simulink library "AtomicLibrary"
PostLoadFcn:
  | PacketBusGenerator; RailCabBusGenerator
(part 2 of 8)

== system AtomicLibrary/UserInterface/Link Layer STATUS.slave ==
  port_in : Inport  Tag=id=_sTPDcPdmEeGH_6eRdlYQdA  Port=1  PortDimensions=-1  DataType=auto  OutDataType=fixdt(1, 16)  OutScaling=2^0  UseBusObject=on  OutDataTypeStr=Inherit: auto
      settings: BusObject=PacketBus
  net_address : Inport  Tag=id=_sTW_QPdmEeGH_6eRdlYQdA  Port=2  PortDimensions=-1  DataType=uint8  OutDataType=fixdt(1, 16)  OutScaling=2^0  OutDataTypeStr=uint8
  receiver_net_address : Inport  Tag=id=_sTXmUPdmEeGH_6eRdlYQdA  Port=3  PortDimensions=-1  DataType=uint8  OutDataType=fixdt(1, 16)  OutScaling=2^0  OutDataTypeStr=uint8
  read_event_queue_in : Inport  Tag=id=_sTQRkPdmEeGH_6eRdlYQdA  Port=4  PortDimensions=-1  DataType=auto  OutDataType=fixdt(1, 16)  OutScaling=2^0  OutDataTypeStr=Inherit: auto
  read_event_param_queue_in : Inport  Tag=id=_sTSt0PdmEeGH_6eRdlYQdA  Port=5  PortDimensions=-1  DataType=auto  OutDataType=fixdt(1, 16)  OutScaling=2^0  OutDataTypeStr=Inherit: auto
  read_event_queue_out : Inport  Tag=id=_sTT78PdmEeGH_6eRdlYQdA  Port=6  PortDimensions=-1  DataType=auto  OutDataType=fixdt(1, 16)  OutScaling=2^0  OutDataTypeStr=Inherit: auto
  read_event_param_queue_out : Inport  Tag=id=_sTUjAPdmEeGH_6eRdlYQdA  Port=7  PortDimensions=-1  DataType=auto  OutDataType=fixdt(1, 16)  OutScaling=2^0  OutDataTypeStr=Inherit: auto
  port_out : Outport  Tag=id=_sTN1UPdmEeGH_6eRdlYQdA  Port=1  PortDimensions=-1  DataType=auto  OutDataType=fixdt(1, 16)  OutScaling=2^0  UseBusObject=on  OutDataTypeStr=Inherit: auto
      settings: BusObject=PacketBus
  write_event_queue_in : Outport  Tag=id=_sTRfsPdmEeGH_6eRdlYQdA  Port=2  PortDimensions=-1  DataType=auto  OutDataType=fixdt(1, 16)  OutScaling=2^0  OutDataTypeStr=Inherit: auto
  write_event_param_queue_in : Outport  Tag=id=_sTSGwPdmEeGH_6eRdlYQdA  Port=3  PortDimensions=-1  DataType=auto  OutDataType=fixdt(1, 16)  OutScaling=2^0  OutDataTypeStr=Inherit: auto
  write_event_queue_out : Outport  Tag=id=_sTVKEPdmEeGH_6eRdlYQdA  Port=4  PortDimensions=-1  DataType=auto  OutDataType=fixdt(1, 16)  OutScaling=2^0  OutDataTypeStr=Inherit: auto
  write_event_param_queue_out : Outport  Tag=id=_sTWYMPdmEeGH_6eRdlYQdA  Port=5  PortDimensions=-1  DataType=auto  OutDataType=fixdt(1, 16)  OutScaling=2^0  OutDataTypeStr=Inherit: auto
  DataLinkLayer : Subsystem  Tag=id=_sTZbgfdmEeGH_6eRdlYQdA
  Bus Selector : BusSelector  OutputSignals=from,to,msg,param,pkgid,time  Tag=id=_sTY0cPdmEeGH_6eRdlYQdA
  Unit Delay1 : UnitDelay  Tag=id=_sTY0cfdmEeGH_6eRdlYQdA  SampleTime=-1
  Unit Delay2 : UnitDelay  Tag=id=_sTZbgPdmEeGH_6eRdlYQdA  SampleTime=-1
  Unit Delay3 : UnitDelay  Tag=id=_sTZbgvdmEeGH_6eRdlYQdA  SampleTime=-1
  Bus Creator : BusCreator  Inputs=6  UseBusObject=on  Tag=id=_sTaCkPdmEeGH_6eRdlYQdA
      settings: BusObject=PacketBus
  Unit Delay4 : UnitDelay  Tag=id=_sTaCkfdmEeGH_6eRdlYQdA  SampleTime=-1
  Terminator : Terminator
      settings: Tag=id=_sTapoPdmEeGH_6eRdlYQdA
  Receive Packet : Stateflow chart  Tag=id=_sTapofdmEeGH_6eRdlYQdA
  Send Packet : Stateflow chart  Tag=id=_sTbQsPdmEeGH_6eRdlYQdA
  wires:
  DataLinkLayer/3(snd_msg_out) -> Bus Creator/3
  DataLinkLayer/8(recv_msg_out) -> Receive Packet/2(packetMsg)
  Send Packet/3(eventQueue) -> Unit Delay1/1
  DataLinkLayer/7(recv_from_out) -> Receive Packet/1(packetFrom)
  Bus Selector/3 -> DataLinkLayer/3(recv_msg_in)
  read_event_param_queue_in/1 -> Receive Packet/5(eventParamQueueIn)
  Receive Packet/3(bufferOverflow) -> Terminator/1
  receiver_net_address/1 -> DataLinkLayer/8(snd_to_in)
  Receive Packet/2(eventParamQueue) -> Unit Delay4/1
  read_event_queue_out/1 -> Send Packet/2(eventQueueIn)
  DataLinkLayer/9(recv_param_out) -> Receive Packet/3(packetParam)
  Send Packet/2(packetParam) -> DataLinkLayer/10(snd_param_in)
  Bus Selector/2 -> DataLinkLayer/2(recv_to_in)
  port_in/1 -> Bus Selector/1
  read_event_param_queue_out/1 -> Send Packet/3(eventParamQueueIn)
  Send Packet/4(eventParamQueue) -> Unit Delay2/1
  Bus Selector/5 -> DataLinkLayer/5(recv_pkgid_in)
  Unit Delay4/1 -> write_event_param_queue_in/1
  read_event_queue_in/1 -> Receive Packet/4(eventQueueIn)
  Bus Selector/4 -> DataLinkLayer/4(recv_param_in)
  DataLinkLayer/2(snd_to_out) -> Bus Creator/2
  Bus Selector/6 -> DataLinkLayer/6(recv_time_in), Send Packet/1(busSizeSignal)
  Receive Packet/1(eventQueue) -> Unit Delay3/1
  DataLinkLayer/6(snd_time_out) -> Bus Creator/6
  Unit Delay1/1 -> write_event_queue_out/1
  DataLinkLayer/1(snd_from_out) -> Bus Creator/1
  DataLinkLayer/5(snd_pkgid_out) -> Bus Creator/5
  net_address/1 -> DataLinkLayer/7(snd_from_in)
  Send Packet/1(packetMsg) -> DataLinkLayer/9(snd_msg_in)
  Bus Creator/1 -> port_out/1  "Outport17"
  Unit Delay3/1 -> write_event_queue_in/1
  Bus Selector/1 -> DataLinkLayer/1(recv_from_in)
  Unit Delay2/1 -> write_event_param_queue_out/1
  DataLinkLayer/4(snd_param_out) -> Bus Creator/4

== system AtomicLibrary/UserInterface/Link Layer HMI_END.master ==
  port_in : Inport  Tag=id=_sdXP0PdmEeGH_6eRdlYQdA  Port=1  PortDimensions=-1  DataType=auto  OutDataType=fixdt(1, 16)  OutScaling=2^0  UseBusObject=on  OutDataTypeStr=Inherit: auto
      settings: BusObject=PacketBus
  net_address : Inport  Tag=id=_sdd9gPdmEeGH_6eRdlYQdA  Port=2  PortDimensions=-1  DataType=uint8  OutDataType=fixdt(1, 16)  OutScaling=2^0  OutDataTypeStr=uint8
  receiver_net_address : Inport  Tag=id=_sdekkPdmEeGH_6eRdlYQdA  Port=3  PortDimensions=-1  DataType=uint8  OutDataType=fixdt(1, 16)  OutScaling=2^0  OutDataTypeStr=uint8
  read_event_queue_in : Inport  Tag=id=_sdX24PdmEeGH_6eRdlYQdA  Port=4  PortDimensions=-1  DataType=auto  OutDataType=fixdt(1, 16)  OutScaling=2^0  OutDataTypeStr=Inherit: auto
  read_event_param_queue_in : Inport  Tag=id=_sdaTIPdmEeGH_6eRdlYQdA  Port=5  PortDimensions=-1  DataType=auto  OutDataType=fixdt(1, 16)  OutScaling=2^0  OutDataTypeStr=Inherit: auto
  read_event_queue_out : Inport  Tag=id=_sda6MPdmEeGH_6eRdlYQdA  Port=6  PortDimensions=-1  DataType=auto  OutDataType=fixdt(1, 16)  OutScaling=2^0  OutDataTypeStr=Inherit: auto
  read_event_param_queue_out : Inport  Tag=id=_sdbhQPdmEeGH_6eRdlYQdA  Port=7  PortDimensions=-1  DataType=auto  OutDataType=fixdt(1, 16)  OutScaling=2^0  OutDataTypeStr=Inherit: auto
  port_out : Outport  Tag=id=_sdWBsfdmEeGH_6eRdlYQdA  Port=1  PortDimensions=-1  DataType=auto  OutDataType=fixdt(1, 16)  OutScaling=2^0  UseBusObject=on  OutDataTypeStr=Inherit: auto
      settings: BusObject=PacketBus
  write_event_queue_in : Outport  Tag=id=_sdYd8PdmEeGH_6eRdlYQdA  Port=2  PortDimensions=-1  DataType=auto  OutDataType=fixdt(1, 16)  OutScaling=2^0  OutDataTypeStr=Inherit: auto
  write_event_param_queue_in : Outport  Tag=id=_sdZFAPdmEeGH_6eRdlYQdA  Port=3  PortDimensions=-1  DataType=auto  OutDataType=fixdt(1, 16)  OutScaling=2^0  OutDataTypeStr=Inherit: auto
  write_event_queue_out : Outport  Tag=id=_sdcIUPdmEeGH_6eRdlYQdA  Port=4  PortDimensions=-1  DataType=auto  OutDataType=fixdt(1, 16)  OutScaling=2^0  OutDataTypeStr=Inherit: auto
  write_event_param_queue_out : Outport  Tag=id=_sddWcPdmEeGH_6eRdlYQdA  Port=5  PortDimensions=-1  DataType=auto  OutDataType=fixdt(1, 16)  OutScaling=2^0  OutDataTypeStr=Inherit: auto
  DataLinkLayer : Subsystem  Tag=id=_sdgZwfdmEeGH_6eRdlYQdA
  Bus Selector : BusSelector  OutputSignals=from,to,msg,param,pkgid,time  Tag=id=_sdfysPdmEeGH_6eRdlYQdA
  Unit Delay1 : UnitDelay  Tag=id=_sdfysfdmEeGH_6eRdlYQdA  SampleTime=-1
  Unit Delay2 : UnitDelay  Tag=id=_sdgZwPdmEeGH_6eRdlYQdA  SampleTime=-1
  Unit Delay3 : UnitDelay  Tag=id=_sdhA0PdmEeGH_6eRdlYQdA  SampleTime=-1
  Bus Creator : BusCreator  Inputs=6  UseBusObject=on  Tag=id=_sdhA0fdmEeGH_6eRdlYQdA
      settings: BusObject=PacketBus
  Unit Delay4 : UnitDelay  Tag=id=_sdhA0vdmEeGH_6eRdlYQdA  SampleTime=-1
  Terminator : Terminator
      settings: Tag=id=_sdhn4PdmEeGH_6eRdlYQdA
  Receive Packet : Stateflow chart  Tag=id=_sdhn4fdmEeGH_6eRdlYQdA
  Send Packet : Stateflow chart  Tag=id=_sdiO8PdmEeGH_6eRdlYQdA
  wires:
  DataLinkLayer/3(snd_msg_out) -> Bus Creator/3
  DataLinkLayer/8(recv_msg_out) -> Receive Packet/2(packetMsg)
  Send Packet/3(eventQueue) -> Unit Delay1/1
  DataLinkLayer/7(recv_from_out) -> Receive Packet/1(packetFrom)
  Bus Selector/3 -> DataLinkLayer/3(recv_msg_in)
  read_event_param_queue_in/1 -> Receive Packet/5(eventParamQueueIn)
  Receive Packet/3(bufferOverflow) -> Terminator/1
  receiver_net_address/1 -> DataLinkLayer/8(snd_to_in)
  Receive Packet/2(eventParamQueue) -> Unit Delay4/1
  read_event_queue_out/1 -> Send Packet/2(eventQueueIn)
  DataLinkLayer/9(recv_param_out) -> Receive Packet/3(packetParam)
  Send Packet/2(packetParam) -> DataLinkLayer/10(snd_param_in)
  Bus Selector/2 -> DataLinkLayer/2(recv_to_in)
  port_in/1 -> Bus Selector/1
  read_event_param_queue_out/1 -> Send Packet/3(eventParamQueueIn)
  Send Packet/4(eventParamQueue) -> Unit Delay2/1
  Bus Selector/5 -> DataLinkLayer/5(recv_pkgid_in)
  Unit Delay4/1 -> write_event_param_queue_in/1
  read_event_queue_in/1 -> Receive Packet/4(eventQueueIn)
  Bus Selector/4 -> DataLinkLayer/4(recv_param_in)
  DataLinkLayer/2(snd_to_out) -> Bus Creator/2
  Bus Selector/6 -> DataLinkLayer/6(recv_time_in), Send Packet/1(busSizeSignal)
  Receive Packet/1(eventQueue) -> Unit Delay3/1
  DataLinkLayer/6(snd_time_out) -> Bus Creator/6
  Unit Delay1/1 -> write_event_queue_out/1
  DataLinkLayer/1(snd_from_out) -> Bus Creator/1
  DataLinkLayer/5(snd_pkgid_out) -> Bus Creator/5
  net_address/1 -> DataLinkLayer/7(snd_from_in)
  Send Packet/1(packetMsg) -> DataLinkLayer/9(snd_msg_in)
  Bus Creator/1 -> port_out/1  "Outport19"
  Unit Delay3/1 -> write_event_queue_in/1
  Bus Selector/1 -> DataLinkLayer/1(recv_from_in)
  Unit Delay2/1 -> write_event_param_queue_out/1
  DataLinkLayer/4(snd_param_out) -> Bus Creator/4

== system AtomicLibrary/TestDelegationSlave/Link Layer delegation_slave ==
  port_in : Inport  Tag=id=_qiNKsPdmEeGH_6eRdlYQdA  Port=1  PortDimensions=-1  DataType=auto  OutDataType=fixdt(1, 16)  OutScaling=2^0  UseBusObject=on  OutDataTypeStr=Inherit: auto
      settings: BusObject=PacketBus
  net_address : Inport  Tag=id=_qiT4YPdmEeGH_6eRdlYQdA  Port=2  PortDimensions=-1  DataType=uint8  OutDataType=fixdt(1, 16)  OutScaling=2^0  OutDataTypeStr=uint8
  receiver_net_address : Inport  Tag=id=_qiVGgPdmEeGH_6eRdlYQdA  Port=3  PortDimensions=-1  DataType=uint8  OutDataType=fixdt(1, 16)  OutScaling=2^0  OutDataTypeStr=uint8
  read_event_queue_in : Inport  Tag=id=_qiNxwPdmEeGH_6eRdlYQdA  Port=4  PortDimensions=-1  DataType=auto  OutDataType=fixdt(1, 16)  OutScaling=2^0  OutDataTypeStr=Inherit: auto
  read_event_param_queue_in : Inport  Tag=id=_qiQOAPdmEeGH_6eRdlYQdA  Port=5  PortDimensions=-1  DataType=auto  OutDataType=fixdt(1, 16)  OutScaling=2^0  OutDataTypeStr=Inherit: auto
  read_event_queue_out : Inport  Tag=id=_qiQ1EPdmEeGH_6eRdlYQdA  Port=6  PortDimensions=-1  DataType=auto  OutDataType=fixdt(1, 16)  OutScaling=2^0  OutDataTypeStr=Inherit: auto
  read_event_param_queue_out : Inport  Tag=id=_qiSDMPdmEeGH_6eRdlYQdA  Port=7  PortDimensions=-1  DataType=auto  OutDataType=fixdt(1, 16)  OutScaling=2^0  OutDataTypeStr=Inherit: auto
  port_out : Outport  Tag=id=_qiL8kfdmEeGH_6eRdlYQdA  Port=1  PortDimensions=-1  DataType=auto  OutDataType=fixdt(1, 16)  OutScaling=2^0  UseBusObject=on  OutDataTypeStr=Inherit: auto
      settings: BusObject=PacketBus
  write_event_queue_in : Outport  Tag=id=_qiO_4PdmEeGH_6eRdlYQdA  Port=2  PortDimensions=-1  DataType=auto  OutDataType=fixdt(1, 16)  OutScaling=2^0  OutDataTypeStr=Inherit: auto
  write_event_param_queue_in : Outport  Tag=id=_qiPm8PdmEeGH_6eRdlYQdA  Port=3  PortDimensions=-1  DataType=auto  OutDataType=fixdt(1, 16)  OutScaling=2^0  OutDataTypeStr=Inherit: auto
  write_event_queue_out : Outport  Tag=id=_qiSqQPdmEeGH_6eRdlYQdA  Port=4  PortDimensions=-1  DataType=auto  OutDataType=fixdt(1, 16)  OutScaling=2^0  OutDataTypeStr=Inherit: auto
  write_event_param_queue_out : Outport  Tag=id=_qiTRUPdmEeGH_6eRdlYQdA  Port=5  PortDimensions=-1  DataType=auto  OutDataType=fixdt(1, 16)  OutScaling=2^0  OutDataTypeStr=Inherit: auto
  DataLinkLayer : Subsystem  Tag=id=_qiW7sfdmEeGH_6eRdlYQdA
  Bus Selector : BusSelector  OutputSignals=from,to,msg,param,pkgid,time  Tag=id=_qiWUoPdmEeGH_6eRdlYQdA
  Unit Delay1 : UnitDelay  Tag=id=_qiWUofdmEeGH_6eRdlYQdA  SampleTime=-1
  Unit Delay2 : UnitDelay  Tag=id=_qiW7sPdmEeGH_6eRdlYQdA  SampleTime=-1
  Unit Delay3 : UnitDelay  Tag=id=_qiXiwPdmEeGH_6eRdlYQdA  SampleTime=-1
  Bus Creator : BusCreator  Inputs=6  UseBusObject=on  Tag=id=_qiYJ0PdmEeGH_6eRdlYQdA
      settings: BusObject=PacketBus
  Unit Delay4 : UnitDelay  Tag=id=_qiYw4PdmEeGH_6eRdlYQdA  SampleTime=-1
  Terminator : Terminator
      settings: Tag=id=_qillMPdmEeGH_6eRdlYQdA
  Receive Packet : Stateflow chart  Tag=id=_qimMQPdmEeGH_6eRdlYQdA
  Send Packet : Stateflow chart  Tag=id=_qimMQfdmEeGH_6eRdlYQdA
  wires:
  DataLinkLayer/3(snd_msg_out) -> Bus Creator/3
  DataLinkLayer/8(recv_msg_out) -> Receive Packet/2(packetMsg)
  Send Packet/3(eventQueue) -> Unit Delay1/1
  DataLinkLayer/7(recv_from_out) -> Receive Packet/1(packetFrom)
  Bus Selector/3 -> DataLinkLayer/3(recv_msg_in)
  read_event_param_queue_in/1 -> Receive Packet/5(eventParamQueueIn)
  Receive Packet/3(bufferOverflow) -> Terminator/1
  receiver_net_address/1 -> DataLinkLayer/8(snd_to_in)
  Receive Packet/2(eventParamQueue) -> Unit Delay4/1
  read_event_queue_out/1 -> Send Packet/2(eventQueueIn)
  DataLinkLayer/9(recv_param_out) -> Receive Packet/3(packetParam)
  Send Packet/2(packetParam) -> DataLinkLayer/10(snd_param_in)
  Bus Selector/2 -> DataLinkLayer/2(recv_to_in)
  port_in/1 -> Bus Selector/1
  read_event_param_queue_out/1 -> Send Packet/3(eventParamQueueIn)
  Send Packet/4(eventParamQueue) -> Unit Delay2/1
  Bus Selector/5 -> DataLinkLayer/5(recv_pkgid_in)
  Unit Delay4/1 -> write_event_param_queue_in/1
  read_event_queue_in/1 -> Receive Packet/4(eventQueueIn)
  Bus Selector/4 -> DataLinkLayer/4(recv_param_in)
  DataLinkLayer/2(snd_to_out) -> Bus Creator/2
  Bus Selector/6 -> DataLinkLayer/6(recv_time_in), Send Packet/1(busSizeSignal)
  Receive Packet/1(eventQueue) -> Unit Delay3/1
  DataLinkLayer/6(snd_time_out) -> Bus Creator/6
  Unit Delay1/1 -> write_event_queue_out/1
  DataLinkLayer/1(snd_from_out) -> Bus Creator/1
  DataLinkLayer/5(snd_pkgid_out) -> Bus Creator/5
  net_address/1 -> DataLinkLayer/7(snd_from_in)
  Send Packet/1(packetMsg) -> DataLinkLayer/9(snd_msg_in)
  Bus Creator/1 -> port_out/1  "Outport21"
  Unit Delay3/1 -> write_event_queue_in/1
  Bus Selector/1 -> DataLinkLayer/1(recv_from_in)
  Unit Delay2/1 -> write_event_param_queue_out/1
  DataLinkLayer/4(snd_param_out) -> Bus Creator/4

== system AtomicLibrary/TestDelegationMaster/Link Layer delegation_master ==
  port_in : Inport  Tag=id=_qrg3sPdmEeGH_6eRdlYQdA  Port=1  PortDimensions=-1  DataType=auto  OutDataType=fixdt(1, 16)  OutScaling=2^0  UseBusObject=on  OutDataTypeStr=Inherit: auto
      settings: BusObject=PacketBus
  net_address : Inport  Tag=id=_qrnlYPdmEeGH_6eRdlYQdA  Port=2  PortDimensions=-1  DataType=uint8  OutDataType=fixdt(1, 16)  OutScaling=2^0  OutDataTypeStr=uint8
  receiver_net_address : Inport  Tag=id=_qroMcPdmEeGH_6eRdlYQdA  Port=3  PortDimensions=-1  DataType=uint8  OutDataType=fixdt(1, 16)  OutScaling=2^0  OutDataTypeStr=uint8
  read_event_queue_in : Inport  Tag=id=_qrhewPdmEeGH_6eRdlYQdA  Port=4  PortDimensions=-1  DataType=auto  OutDataType=fixdt(1, 16)  OutScaling=2^0  OutDataTypeStr=Inherit: auto
  read_event_param_queue_in : Inport  Tag=id=_qrj7APdmEeGH_6eRdlYQdA  Port=5  PortDimensions=-1  DataType=auto  OutDataType=fixdt(1, 16)  OutScaling=2^0  OutDataTypeStr=Inherit: auto
  read_event_queue_out : Inport  Tag=id=_qrkiEPdmEeGH_6eRdlYQdA  Port=6  PortDimensions=-1  DataType=auto  OutDataType=fixdt(1, 16)  OutScaling=2^0  OutDataTypeStr=Inherit: auto
  read_event_param_queue_out : Inport  Tag=id=_qrlwMPdmEeGH_6eRdlYQdA  Port=7  PortDimensions=-1  DataType=auto  OutDataType=fixdt(1, 16)  OutScaling=2^0  OutDataTypeStr=Inherit: auto
  port_out : Outport  Tag=id=_qrgQofdmEeGH_6eRdlYQdA  Port=1  PortDimensions=-1  DataType=auto  OutDataType=fixdt(1, 16)  OutScaling=2^0  UseBusObject=on  OutDataTypeStr=Inherit: auto
      settings: BusObject=PacketBus
  write_event_queue_in : Outport  Tag=id=_qriF0PdmEeGH_6eRdlYQdA  Port=2  PortDimensions=-1  DataType=auto  OutDataType=fixdt(1, 16)  OutScaling=2^0  OutDataTypeStr=Inherit: auto
  write_event_param_queue_in : Outport  Tag=id=_qrjT8PdmEeGH_6eRdlYQdA  Port=3  PortDimensions=-1  DataType=auto  OutDataType=fixdt(1, 16)  OutScaling=2^0  OutDataTypeStr=Inherit: auto
  write_event_queue_out : Outport  Tag=id=_qrmXQPdmEeGH_6eRdlYQdA  Port=4  PortDimensions=-1  DataType=auto  OutDataType=fixdt(1, 16)  OutScaling=2^0  OutDataTypeStr=Inherit: auto
  write_event_param_queue_out : Outport  Tag=id=_qrm-UPdmEeGH_6eRdlYQdA  Port=5  PortDimensions=-1  DataType=auto  OutDataType=fixdt(1, 16)  OutScaling=2^0  OutDataTypeStr=Inherit: auto
  DataLinkLayer : Subsystem  Tag=id=_qrpakvdmEeGH_6eRdlYQdA
  Bus Selector : BusSelector  OutputSignals=from,to,msg,param,pkgid,time  Tag=id=_qrozgPdmEeGH_6eRdlYQdA
  Unit Delay1 : UnitDelay  Tag=id=_qrpakPdmEeGH_6eRdlYQdA  SampleTime=-1
  Unit Delay2 : UnitDelay  Tag=id=_qrpakfdmEeGH_6eRdlYQdA  SampleTime=-1
  Unit Delay3 : UnitDelay  Tag=id=_qrqBoPdmEeGH_6eRdlYQdA  SampleTime=-1
  Bus Creator : BusCreator  Inputs=6  UseBusObject=on  Tag=id=_qrqBofdmEeGH_6eRdlYQdA
      settings: BusObject=PacketBus
  Unit Delay4 : UnitDelay  Tag=id=_qrqosPdmEeGH_6eRdlYQdA  SampleTime=-1
  Terminator : Terminator
      settings: Tag=id=_qrqosfdmEeGH_6eRdlYQdA
  Receive Packet : Stateflow chart  Tag=id=_qrrPwPdmEeGH_6eRdlYQdA
  Send Packet : Stateflow chart  Tag=id=_qrrPwfdmEeGH_6eRdlYQdA
  wires:
  DataLinkLayer/3(snd_msg_out) -> Bus Creator/3
  DataLinkLayer/8(recv_msg_out) -> Receive Packet/2(packetMsg)
  Send Packet/3(eventQueue) -> Unit Delay1/1
  DataLinkLayer/7(recv_from_out) -> Receive Packet/1(packetFrom)
  Bus Selector/3 -> DataLinkLayer/3(recv_msg_in)
  read_event_param_queue_in/1 -> Receive Packet/5(eventParamQueueIn)
  Receive Packet/3(bufferOverflow) -> Terminator/1
  receiver_net_address/1 -> DataLinkLayer/8(snd_to_in)
  Receive Packet/2(eventParamQueue) -> Unit Delay4/1
  read_event_queue_out/1 -> Send Packet/2(eventQueueIn)
  DataLinkLayer/9(recv_param_out) -> Receive Packet/3(packetParam)
  Send Packet/2(packetParam) -> DataLinkLayer/10(snd_param_in)
  Bus Selector/2 -> DataLinkLayer/2(recv_to_in)
  port_in/1 -> Bus Selector/1
  read_event_param_queue_out/1 -> Send Packet/3(eventParamQueueIn)
  Send Packet/4(eventParamQueue) -> Unit Delay2/1
  Bus Selector/5 -> DataLinkLayer/5(recv_pkgid_in)
  Unit Delay4/1 -> write_event_param_queue_in/1
  read_event_queue_in/1 -> Receive Packet/4(eventQueueIn)
  Bus Selector/4 -> DataLinkLayer/4(recv_param_in)
  DataLinkLayer/2(snd_to_out) -> Bus Creator/2
  Bus Selector/6 -> DataLinkLayer/6(recv_time_in), Send Packet/1(busSizeSignal)
  Receive Packet/1(eventQueue) -> Unit Delay3/1
  DataLinkLayer/6(snd_time_out) -> Bus Creator/6
  Unit Delay1/1 -> write_event_queue_out/1
  DataLinkLayer/1(snd_from_out) -> Bus Creator/1
  DataLinkLayer/5(snd_pkgid_out) -> Bus Creator/5
  net_address/1 -> DataLinkLayer/7(snd_from_in)
  Send Packet/1(packetMsg) -> DataLinkLayer/9(snd_msg_in)
  Bus Creator/1 -> port_out/1  "Outport23"
  Unit Delay3/1 -> write_event_queue_in/1
  Bus Selector/1 -> DataLinkLayer/1(recv_from_in)
  Unit Delay2/1 -> write_event_param_queue_out/1
  DataLinkLayer/4(snd_param_out) -> Bus Creator/4

== system AtomicLibrary/TestEventListenerSlave/Link Layer eventListener_slave ==
  port_in : Inport  Tag=id=_q0oXcPdmEeGH_6eRdlYQdA  Port=1  PortDimensions=-1  DataType=auto  OutDataType=fixdt(1, 16)  OutScaling=2^0  UseBusObject=on  OutDataTypeStr=Inherit: auto
      settings: BusObject=PacketBus
  net_address : Inport  Tag=id=_q0vsMPdmEeGH_6eRdlYQdA  Port=2  PortDimensions=-1  DataType=uint8  OutDataType=fixdt(1, 16)  OutScaling=2^0  OutDataTypeStr=uint8
  receiver_net_address : Inport  Tag=id=_q0vsMfdmEeGH_6eRdlYQdA  Port=3  PortDimensions=-1  DataType=uint8  OutDataType=fixdt(1, 16)  OutScaling=2^0  OutDataTypeStr=uint8
  read_event_queue_in : Inport  Tag=id=_q0o-gPdmEeGH_6eRdlYQdA  Port=4  PortDimensions=-1  DataType=auto  OutDataType=fixdt(1, 16)  OutScaling=2^0  OutDataTypeStr=Inherit: auto
  read_event_param_queue_in : Inport  Tag=id=_q0rawPdmEeGH_6eRdlYQdA  Port=5  PortDimensions=-1  DataType=auto  OutDataType=fixdt(1, 16)  OutScaling=2^0  OutDataTypeStr=Inherit: auto
  read_event_queue_out : Inport  Tag=id=_q0so4PdmEeGH_6eRdlYQdA  Port=6  PortDimensions=-1  DataType=auto  OutDataType=fixdt(1, 16)  OutScaling=2^0  OutDataTypeStr=Inherit: auto
  read_event_param_queue_out : Inport  Tag=id=_q0tP8PdmEeGH_6eRdlYQdA  Port=7  PortDimensions=-1  DataType=auto  OutDataType=fixdt(1, 16)  OutScaling=2^0  OutDataTypeStr=Inherit: auto
  port_out : Outport  Tag=id=_q0nwYfdmEeGH_6eRdlYQdA  Port=1  PortDimensions=-1  DataType=auto  OutDataType=fixdt(1, 16)  OutScaling=2^0  UseBusObject=on  OutDataTypeStr=Inherit: auto
      settings: BusObject=PacketBus
  write_event_queue_in : Outport  Tag=id=_q0plkPdmEeGH_6eRdlYQdA  Port=2  PortDimensions=-1  DataType=auto  OutDataType=fixdt(1, 16)  OutScaling=2^0  OutDataTypeStr=Inherit: auto
  write_event_param_queue_in : Outport  Tag=id=_q0qzsPdmEeGH_6eRdlYQdA  Port=3  PortDimensions=-1  DataType=auto  OutDataType=fixdt(1, 16)  OutScaling=2^0  OutDataTypeStr=Inherit: auto
  write_event_queue_out : Outport  Tag=id=_q0t3APdmEeGH_6eRdlYQdA  Port=4  PortDimensions=-1  DataType=auto  OutDataType=fixdt(1, 16)  OutScaling=2^0  OutDataTypeStr=Inherit: auto
  write_event_param_queue_out : Outport  Tag=id=_q0ueEPdmEeGH_6eRdlYQdA  Port=5  PortDimensions=-1  DataType=auto  OutDataType=fixdt(1, 16)  OutScaling=2^0  OutDataTypeStr=Inherit: auto
  DataLinkLayer : Subsystem  Tag=id=_q0xhYPdmEeGH_6eRdlYQdA
  Bus Selector : BusSelector  OutputSignals=from,to,msg,param,pkgid,time  Tag=id=_q0w6UPdmEeGH_6eRdlYQdA
  Unit Delay1 : UnitDelay  Tag=id=_q0w6UfdmEeGH_6eRdlYQdA  SampleTime=-1
  Unit Delay2 : UnitDelay  Tag=id=_q0w6UvdmEeGH_6eRdlYQdA  SampleTime=-1
  Unit Delay3 : UnitDelay  Tag=id=_q0xhYfdmEeGH_6eRdlYQdA  SampleTime=-1
  Bus Creator : BusCreator  Inputs=6  UseBusObject=on  Tag=id=_q0yIcPdmEeGH_6eRdlYQdA
      settings: BusObject=PacketBus
  Unit Delay4 : UnitDelay  Tag=id=_q0yIcfdmEeGH_6eRdlYQdA  SampleTime=-1
  Terminator : Terminator
      settings: Tag=id=_q0yIcvdmEeGH_6eRdlYQdA
  Receive Packet : Stateflow chart  Tag=id=_q0yvgPdmEeGH_6eRdlYQdA
  Send Packet : Stateflow chart  Tag=id=_q0zWkPdmEeGH_6eRdlYQdA
  wires:
  DataLinkLayer/3(snd_msg_out) -> Bus Creator/3
  DataLinkLayer/8(recv_msg_out) -> Receive Packet/2(packetMsg)
  Send Packet/3(eventQueue) -> Unit Delay1/1
  DataLinkLayer/7(recv_from_out) -> Receive Packet/1(packetFrom)
  Bus Selector/3 -> DataLinkLayer/3(recv_msg_in)
  read_event_param_queue_in/1 -> Receive Packet/5(eventParamQueueIn)
  Receive Packet/3(bufferOverflow) -> Terminator/1
  receiver_net_address/1 -> DataLinkLayer/8(snd_to_in)
  Receive Packet/2(eventParamQueue) -> Unit Delay4/1
  read_event_queue_out/1 -> Send Packet/2(eventQueueIn)
  DataLinkLayer/9(recv_param_out) -> Receive Packet/3(packetParam)
  Send Packet/2(packetParam) -> DataLinkLayer/10(snd_param_in)
  Bus Selector/2 -> DataLinkLayer/2(recv_to_in)
  port_in/1 -> Bus Selector/1
  read_event_param_queue_out/1 -> Send Packet/3(eventParamQueueIn)
  Send Packet/4(eventParamQueue) -> Unit Delay2/1
  Bus Selector/5 -> DataLinkLayer/5(recv_pkgid_in)
  Unit Delay4/1 -> write_event_param_queue_in/1
  read_event_queue_in/1 -> Receive Packet/4(eventQueueIn)
  Bus Selector/4 -> DataLinkLayer/4(recv_param_in)
  DataLinkLayer/2(snd_to_out) -> Bus Creator/2
  Bus Selector/6 -> DataLinkLayer/6(recv_time_in), Send Packet/1(busSizeSignal)
  Receive Packet/1(eventQueue) -> Unit Delay3/1
  DataLinkLayer/6(snd_time_out) -> Bus Creator/6
  Unit Delay1/1 -> write_event_queue_out/1
  DataLinkLayer/1(snd_from_out) -> Bus Creator/1
  DataLinkLayer/5(snd_pkgid_out) -> Bus Creator/5
  net_address/1 -> DataLinkLayer/7(snd_from_in)
  Send Packet/1(packetMsg) -> DataLinkLayer/9(snd_msg_in)
  Bus Creator/1 -> port_out/1  "Outport25"
  Unit Delay3/1 -> write_event_queue_in/1
  Bus Selector/1 -> DataLinkLayer/1(recv_from_in)
  Unit Delay2/1 -> write_event_param_queue_out/1
  DataLinkLayer/4(snd_param_out) -> Bus Creator/4

== system AtomicLibrary/TestEventListenerMaster/Link Layer eventListener_master ==
  port_in : Inport  Tag=id=_q93L8PdmEeGH_6eRdlYQdA  Port=1  PortDimensions=-1  DataType=auto  OutDataType=fixdt(1, 16)  OutScaling=2^0  UseBusObject=on  OutDataTypeStr=Inherit: auto
      settings: BusObject=PacketBus
  net_address : Inport  Tag=id=_q99SkPdmEeGH_6eRdlYQdA  Port=2  PortDimensions=-1  DataType=uint8  OutDataType=fixdt(1, 16)  OutScaling=2^0  OutDataTypeStr=uint8
  receiver_net_address : Inport  Tag=id=_q995oPdmEeGH_6eRdlYQdA  Port=3  PortDimensions=-1  DataType=uint8  OutDataType=fixdt(1, 16)  OutScaling=2^0  OutDataTypeStr=uint8
  read_event_queue_in : Inport  Tag=id=_q93zAPdmEeGH_6eRdlYQdA  Port=4  PortDimensions=-1  DataType=auto  OutDataType=fixdt(1, 16)  OutScaling=2^0  OutDataTypeStr=Inherit: auto
  read_event_param_queue_in : Inport  Tag=id=_q96PQPdmEeGH_6eRdlYQdA  Port=5  PortDimensions=-1  DataType=auto  OutDataType=fixdt(1, 16)  OutScaling=2^0  OutDataTypeStr=Inherit: auto
  read_event_queue_out : Inport  Tag=id=_q962UPdmEeGH_6eRdlYQdA  Port=6  PortDimensions=-1  DataType=auto  OutDataType=fixdt(1, 16)  OutScaling=2^0  OutDataTypeStr=Inherit: auto
  read_event_param_queue_out : Inport  Tag=id=_q97dYPdmEeGH_6eRdlYQdA  Port=7  PortDimensions=-1  DataType=auto  OutDataType=fixdt(1, 16)  OutScaling=2^0  OutDataTypeStr=Inherit: auto
  port_out : Outport  Tag=id=_q92k4fdmEeGH_6eRdlYQdA  Port=1  PortDimensions=-1  DataType=auto  OutDataType=fixdt(1, 16)  OutScaling=2^0  UseBusObject=on  OutDataTypeStr=Inherit: auto
      settings: BusObject=PacketBus
  write_event_queue_in : Outport  Tag=id=_q94aEPdmEeGH_6eRdlYQdA  Port=2  PortDimensions=-1  DataType=auto  OutDataType=fixdt(1, 16)  OutScaling=2^0  OutDataTypeStr=Inherit: auto
  write_event_param_queue_in : Outport  Tag=id=_q95oMPdmEeGH_6eRdlYQdA  Port=3  PortDimensions=-1  DataType=auto  OutDataType=fixdt(1, 16)  OutScaling=2^0  OutDataTypeStr=Inherit: auto
  write_event_queue_out : Outport  Tag=id=_q98EcPdmEeGH_6eRdlYQdA  Port=4  PortDimensions=-1  DataType=auto  OutDataType=fixdt(1, 16)  OutScaling=2^0  OutDataTypeStr=Inherit: auto
  write_event_param_queue_out : Outport  Tag=id=_q98rgPdmEeGH_6eRdlYQdA  Port=5  PortDimensions=-1  DataType=auto  OutDataType=fixdt(1, 16)  OutScaling=2^0  OutDataTypeStr=Inherit: auto
  DataLinkLayer : Subsystem  Tag=id=_q9_HwvdmEeGH_6eRdlYQdA
  Bus Selector : BusSelector  OutputSignals=from,to,msg,param,pkgid,time  Tag=id=_q9-gsPdmEeGH_6eRdlYQdA
  Unit Delay1 : UnitDelay  Tag=id=_q9_HwPdmEeGH_6eRdlYQdA  SampleTime=-1
  Unit Delay2 : UnitDelay  Tag=id=_q9_HwfdmEeGH_6eRdlYQdA  SampleTime=-1
  Unit Delay3 : UnitDelay  Tag=id=_q9_u0PdmEeGH_6eRdlYQdA  SampleTime=-1
  Bus Creator : BusCreator  Inputs=6  UseBusObject=on  Tag=id=_q9_u0fdmEeGH_6eRdlYQdA
      settings: BusObject=PacketBus
  Unit Delay4 : UnitDelay  Tag=id=_q-AV4PdmEeGH_6eRdlYQdA  SampleTime=-1
  Terminator : Terminator
      settings: Tag=id=_q-AV4fdmEeGH_6eRdlYQdA
  Receive Packet : Stateflow chart  Tag=id=_q-AV4vdmEeGH_6eRdlYQdA
  Send Packet : Stateflow chart  Tag=id=_q-A88PdmEeGH_6eRdlYQdA
  wires:
  DataLinkLayer/3(snd_msg_out) -> Bus Creator/3
  DataLinkLayer/8(recv_msg_out) -> Receive Packet/2(packetMsg)
  Send Packet/3(eventQueue) -> Unit Delay1/1
  DataLinkLayer/7(recv_from_out) -> Receive Packet/1(packetFrom)
  Bus Selector/3 -> DataLinkLayer/3(recv_msg_in)
  read_event_param_queue_in/1 -> Receive Packet/5(eventParamQueueIn)
  Receive Packet/3(bufferOverflow) -> Terminator/1
  receiver_net_address/1 -> DataLinkLayer/8(snd_to_in)
  Receive Packet/2(eventParamQueue) -> Unit Delay4/1
  read_event_queue_out/1 -> Send Packet/2(eventQueueIn)
  DataLinkLayer/9(recv_param_out) -> Receive Packet/3(packetParam)
  Send Packet/2(packetParam) -> DataLinkLayer/10(snd_param_in)
  Bus Selector/2 -> DataLinkLayer/2(recv_to_in)
  port_in/1 -> Bus Selector/1
  read_event_param_queue_out/1 -> Send Packet/3(eventParamQueueIn)
  Send Packet/4(eventParamQueue) -> Unit Delay2/1
  Bus Selector/5 -> DataLinkLayer/5(recv_pkgid_in)
  Unit Delay4/1 -> write_event_param_queue_in/1
  read_event_queue_in/1 -> Receive Packet/4(eventQueueIn)
  Bus Selector/4 -> DataLinkLayer/4(recv_param_in)
  DataLinkLayer/2(snd_to_out) -> Bus Creator/2
  Bus Selector/6 -> DataLinkLayer/6(recv_time_in), Send Packet/1(busSizeSignal)
  Receive Packet/1(eventQueue) -> Unit Delay3/1
  DataLinkLayer/6(snd_time_out) -> Bus Creator/6
  Unit Delay1/1 -> write_event_queue_out/1
  DataLinkLayer/1(snd_from_out) -> Bus Creator/1
  DataLinkLayer/5(snd_pkgid_out) -> Bus Creator/5
  net_address/1 -> DataLinkLayer/7(snd_from_in)
  Send Packet/1(packetMsg) -> DataLinkLayer/9(snd_msg_in)
  Bus Creator/1 -> port_out/1  "Outport27"
  Unit Delay3/1 -> write_event_queue_in/1
  Bus Selector/1 -> DataLinkLayer/1(recv_from_in)
  Unit Delay2/1 -> write_event_param_queue_out/1
  DataLinkLayer/4(snd_param_out) -> Bus Creator/4

== system AtomicLibrary/TestTurnTransmission/Link Layer turn_transmission_partner ==
  port_in : Inport  Tag=id=_rGp7kPdmEeGH_6eRdlYQdA  Port=1  PortDimensions=-1  DataType=auto  OutDataType=fixdt(1, 16)  OutScaling=2^0  UseBusObject=on  OutDataTypeStr=Inherit: auto
      settings: BusObject=PacketBus
  net_address : Inport  Tag=id=_rGvbIPdmEeGH_6eRdlYQdA  Port=2  PortDimensions=-1  DataType=uint8  OutDataType=fixdt(1, 16)  OutScaling=2^0  OutDataTypeStr=uint8
  receiver_net_address : Inport  Tag=id=_rGwCMPdmEeGH_6eRdlYQdA  Port=3  PortDimensions=-1  DataType=uint8  OutDataType=fixdt(1, 16)  OutScaling=2^0  OutDataTypeStr=uint8
  read_event_queue_in : Inport  Tag=id=_rGqioPdmEeGH_6eRdlYQdA  Port=4  PortDimensions=-1  DataType=auto  OutDataType=fixdt(1, 16)  OutScaling=2^0  OutDataTypeStr=Inherit: auto
  read_event_param_queue_in : Inport  Tag=id=_rGsX0PdmEeGH_6eRdlYQdA  Port=5  PortDimensions=-1  DataType=auto  OutDataType=fixdt(1, 16)  OutScaling=2^0  OutDataTypeStr=Inherit: auto
  read_event_queue_out : Inport  Tag=id=_rGs-4PdmEeGH_6eRdlYQdA  Port=6  PortDimensions=-1  DataType=auto  OutDataType=fixdt(1, 16)  OutScaling=2^0  OutDataTypeStr=Inherit: auto
  read_event_param_queue_out : Inport  Tag=id=_rGtl8PdmEeGH_6eRdlYQdA  Port=7  PortDimensions=-1  DataType=auto  OutDataType=fixdt(1, 16)  OutScaling=2^0  OutDataTypeStr=Inherit: auto
  port_out : Outport  Tag=id=_rGpUgPdmEeGH_6eRdlYQdA  Port=1  PortDimensions=-1  DataType=auto  OutDataType=fixdt(1, 16)  OutScaling=2^0  UseBusObject=on  OutDataTypeStr=Inherit: auto
      settings: BusObject=PacketBus
  write_event_queue_in : Outport  Tag=id=_rGrJsPdmEeGH_6eRdlYQdA  Port=2  PortDimensions=-1  DataType=auto  OutDataType=fixdt(1, 16)  OutScaling=2^0  OutDataTypeStr=Inherit: auto
  write_event_param_queue_in : Outport  Tag=id=_rGrwwPdmEeGH_6eRdlYQdA  Port=3  PortDimensions=-1  DataType=auto  OutDataType=fixdt(1, 16)  OutScaling=2^0  OutDataTypeStr=Inherit: auto
  write_event_queue_out : Outport  Tag=id=_rGuNAPdmEeGH_6eRdlYQdA  Port=4  PortDimensions=-1  DataType=auto  OutDataType=fixdt(1, 16)  OutScaling=2^0  OutDataTypeStr=Inherit: auto
  write_event_param_queue_out : Outport  Tag=id=_rGu0EPdmEeGH_6eRdlYQdA  Port=5  PortDimensions=-1  DataType=auto  OutDataType=fixdt(1, 16)  OutScaling=2^0  OutDataTypeStr=Inherit: auto
  DataLinkLayer : Subsystem  Tag=id=_rGxQUvdmEeGH_6eRdlYQdA
  Bus Selector : BusSelector  OutputSignals=from,to,msg,param,pkgid,time  Tag=id=_rGwpQPdmEeGH_6eRdlYQdA
  Unit Delay1 : UnitDelay  Tag=id=_rGxQUPdmEeGH_6eRdlYQdA  SampleTime=-1
  Unit Delay2 : UnitDelay  Tag=id=_rGxQUfdmEeGH_6eRdlYQdA  SampleTime=-1
  Unit Delay3 : UnitDelay  Tag=id=_rGx3YPdmEeGH_6eRdlYQdA  SampleTime=-1
  Bus Creator : BusCreator  Inputs=6  UseBusObject=on  Tag=id=_rGx3YfdmEeGH_6eRdlYQdA
      settings: BusObject=PacketBus
  Unit Delay4 : UnitDelay  Tag=id=_rGyecPdmEeGH_6eRdlYQdA  SampleTime=-1
  Terminator : Terminator
      settings: Tag=id=_rGyecfdmEeGH_6eRdlYQdA
  Receive Packet : Stateflow chart  Tag=id=_rGzFgPdmEeGH_6eRdlYQdA
  Send Packet : Stateflow chart  Tag=id=_rGzFgfdmEeGH_6eRdlYQdA
  wires:
  DataLinkLayer/3(snd_msg_out) -> Bus Creator/3
  DataLinkLayer/8(recv_msg_out) -> Receive Packet/2(packetMsg)
  Send Packet/3(eventQueue) -> Unit Delay1/1
  DataLinkLayer/7(recv_from_out) -> Receive Packet/1(packetFrom)
  Bus Selector/3 -> DataLinkLayer/3(recv_msg_in)
  read_event_param_queue_in/1 -> Receive Packet/5(eventParamQueueIn)
  Receive Packet/3(bufferOverflow) -> Terminator/1
  receiver_net_address/1 -> DataLinkLayer/8(snd_to_in)
  Receive Packet/2(eventParamQueue) -> Unit Delay4/1
  read_event_queue_out/1 -> Send Packet/2(eventQueueIn)
  DataLinkLayer/9(recv_param_out) -> Receive Packet/3(packetParam)
  Send Packet/2(packetParam) -> DataLinkLayer/10(snd_param_in)
  Bus Selector/2 -> DataLinkLayer/2(recv_to_in)
  port_in/1 -> Bus Selector/1
  read_event_param_queue_out/1 -> Send Packet/3(eventParamQueueIn)
  Send Packet/4(eventParamQueue) -> Unit Delay2/1
  Bus Selector/5 -> DataLinkLayer/5(recv_pkgid_in)
  Unit Delay4/1 -> write_event_param_queue_in/1
  read_event_queue_in/1 -> Receive Packet/4(eventQueueIn)
  Bus Selector/4 -> DataLinkLayer/4(recv_param_in)
  DataLinkLayer/2(snd_to_out) -> Bus Creator/2
  Bus Selector/6 -> DataLinkLayer/6(recv_time_in), Send Packet/1(busSizeSignal)
  Receive Packet/1(eventQueue) -> Unit Delay3/1
  DataLinkLayer/6(snd_time_out) -> Bus Creator/6
  Unit Delay1/1 -> write_event_queue_out/1
  DataLinkLayer/1(snd_from_out) -> Bus Creator/1
  DataLinkLayer/5(snd_pkgid_out) -> Bus Creator/5
  net_address/1 -> DataLinkLayer/7(snd_from_in)
  Send Packet/1(packetMsg) -> DataLinkLayer/9(snd_msg_in)
  Bus Creator/1 -> port_out/1  "Outport29"
  Unit Delay3/1 -> write_event_queue_in/1
  Bus Selector/1 -> DataLinkLayer/1(recv_from_in)
  Unit Delay2/1 -> write_event_param_queue_out/1
  DataLinkLayer/4(snd_param_out) -> Bus Creator/4

== system AtomicLibrary/TestRequestInformationProvider/Link Layer requestinformation_provider ==
  port_in : Inport  Tag=id=_rPz3kPdmEeGH_6eRdlYQdA  Port=1  PortDimensions=-1  DataType=auto  OutDataType=fixdt(1, 16)  OutScaling=2^0  UseBusObject=on  OutDataTypeStr=Inherit: auto
      settings: BusObject=PacketBus
  net_address : Inport  Tag=id=_rP7zYPdmEeGH_6eRdlYQdA  Port=2  PortDimensions=-1  DataType=uint8  OutDataType=fixdt(1, 16)  OutScaling=2^0  OutDataTypeStr=uint8
  receiver_net_address : Inport  Tag=id=_rP8acPdmEeGH_6eRdlYQdA  Port=3  PortDimensions=-1  DataType=uint8  OutDataType=fixdt(1, 16)  OutScaling=2^0  OutDataTypeStr=uint8
  read_event_queue_in : Inport  Tag=id=_rP1FsPdmEeGH_6eRdlYQdA  Port=4  PortDimensions=-1  DataType=auto  OutDataType=fixdt(1, 16)  OutScaling=2^0  OutDataTypeStr=Inherit: auto
  read_event_param_queue_in : Inport  Tag=id=_rP4JAPdmEeGH_6eRdlYQdA  Port=5  PortDimensions=-1  DataType=auto  OutDataType=fixdt(1, 16)  OutScaling=2^0  OutDataTypeStr=Inherit: auto
  read_event_queue_out : Inport  Tag=id=_rP4wEPdmEeGH_6eRdlYQdA  Port=6  PortDimensions=-1  DataType=auto  OutDataType=fixdt(1, 16)  OutScaling=2^0  OutDataTypeStr=Inherit: auto
  read_event_param_queue_out : Inport  Tag=id=_rP5XIPdmEeGH_6eRdlYQdA  Port=7  PortDimensions=-1  DataType=auto  OutDataType=fixdt(1, 16)  OutScaling=2^0  OutDataTypeStr=Inherit: auto
  port_out : Outport  Tag=id=_rPzQgPdmEeGH_6eRdlYQdA  Port=1  PortDimensions=-1  DataType=auto  OutDataType=fixdt(1, 16)  OutScaling=2^0  UseBusObject=on  OutDataTypeStr=Inherit: auto
      settings: BusObject=PacketBus
  write_event_queue_in : Outport  Tag=id=_rP2T0PdmEeGH_6eRdlYQdA  Port=2  PortDimensions=-1  DataType=auto  OutDataType=fixdt(1, 16)  OutScaling=2^0  OutDataTypeStr=Inherit: auto
  write_event_param_queue_in : Outport  Tag=id=_rP264PdmEeGH_6eRdlYQdA  Port=3  PortDimensions=-1  DataType=auto  OutDataType=fixdt(1, 16)  OutScaling=2^0  OutDataTypeStr=Inherit: auto
  write_event_queue_out : Outport  Tag=id=_rP5-MPdmEeGH_6eRdlYQdA  Port=4  PortDimensions=-1  DataType=auto  OutDataType=fixdt(1, 16)  OutScaling=2^0  OutDataTypeStr=Inherit: auto
  write_event_param_queue_out : Outport  Tag=id=_rP7MUPdmEeGH_6eRdlYQdA  Port=5  PortDimensions=-1  DataType=auto  OutDataType=fixdt(1, 16)  OutScaling=2^0  OutDataTypeStr=Inherit: auto
  DataLinkLayer : Subsystem  Tag=id=_rP9okfdmEeGH_6eRdlYQdA
  Bus Selector : BusSelector  OutputSignals=from,to,msg,param,pkgid,time  Tag=id=_rP9BgPdmEeGH_6eRdlYQdA
  Unit Delay1 : UnitDelay  Tag=id=_rP9BgfdmEeGH_6eRdlYQdA  SampleTime=-1
  Unit Delay2 : UnitDelay  Tag=id=_rP9okPdmEeGH_6eRdlYQdA  SampleTime=-1
  Unit Delay3 : UnitDelay  Tag=id=_rP-PoPdmEeGH_6eRdlYQdA  SampleTime=-1
  Bus Creator : BusCreator  Inputs=6  UseBusObject=on  Tag=id=_rP-PofdmEeGH_6eRdlYQdA
      settings: BusObject=PacketBus
  Unit Delay4 : UnitDelay  Tag=id=_rP-PovdmEeGH_6eRdlYQdA  SampleTime=-1
  Terminator : Terminator
      settings: Tag=id=_rP-2sPdmEeGH_6eRdlYQdA
  Receive Packet : Stateflow chart  Tag=id=_rP-2sfdmEeGH_6eRdlYQdA
  Send Packet : Stateflow chart  Tag=id=_rP_dwPdmEeGH_6eRdlYQdA
  wires:
  DataLinkLayer/3(snd_msg_out) -> Bus Creator/3
  DataLinkLayer/8(recv_msg_out) -> Receive Packet/2(packetMsg)
  Send Packet/3(eventQueue) -> Unit Delay1/1
  DataLinkLayer/7(recv_from_out) -> Receive Packet/1(packetFrom)
  Bus Selector/3 -> DataLinkLayer/3(recv_msg_in)
  read_event_param_queue_in/1 -> Receive Packet/5(eventParamQueueIn)
  Receive Packet/3(bufferOverflow) -> Terminator/1
  receiver_net_address/1 -> DataLinkLayer/8(snd_to_in)
  Receive Packet/2(eventParamQueue) -> Unit Delay4/1
  read_event_queue_out/1 -> Send Packet/2(eventQueueIn)
  DataLinkLayer/9(recv_param_out) -> Receive Packet/3(packetParam)
  Send Packet/2(packetParam) -> DataLinkLayer/10(snd_param_in)
  Bus Selector/2 -> DataLinkLayer/2(recv_to_in)
  port_in/1 -> Bus Selector/1
  read_event_param_queue_out/1 -> Send Packet/3(eventParamQueueIn)
  Send Packet/4(eventParamQueue) -> Unit Delay2/1
  Bus Selector/5 -> DataLinkLayer/5(recv_pkgid_in)
  Unit Delay4/1 -> write_event_param_queue_in/1
  read_event_queue_in/1 -> Receive Packet/4(eventQueueIn)
  Bus Selector/4 -> DataLinkLayer/4(recv_param_in)
  DataLinkLayer/2(snd_to_out) -> Bus Creator/2
  Bus Selector/6 -> DataLinkLayer/6(recv_time_in), Send Packet/1(busSizeSignal)
  Receive Packet/1(eventQueue) -> Unit Delay3/1
  DataLinkLayer/6(snd_time_out) -> Bus Creator/6
  Unit Delay1/1 -> write_event_queue_out/1
  DataLinkLayer/1(snd_from_out) -> Bus Creator/1
  DataLinkLayer/5(snd_pkgid_out) -> Bus Creator/5
  net_address/1 -> DataLinkLayer/7(snd_from_in)
  Send Packet/1(packetMsg) -> DataLinkLayer/9(snd_msg_in)
  Bus Creator/1 -> port_out/1  "Outport31"
  Unit Delay3/1 -> write_event_queue_in/1
  Bus Selector/1 -> DataLinkLayer/1(recv_from_in)
  Unit Delay2/1 -> write_event_param_queue_out/1
  DataLinkLayer/4(snd_param_out) -> Bus Creator/4

== system AtomicLibrary/TestRequestInformaitonUser/Link Layer requestinformation_user ==
  port_in : Inport  Tag=id=_rYOzwPdmEeGH_6eRdlYQdA  Port=1  PortDimensions=-1  DataType=auto  OutDataType=fixdt(1, 16)  OutScaling=2^0  UseBusObject=on  OutDataTypeStr=Inherit: auto
      settings: BusObject=PacketBus
  net_address : Inport  Tag=id=_rYWvkPdmEeGH_6eRdlYQdA  Port=2  PortDimensions=-1  DataType=uint8  OutDataType=fixdt(1, 16)  OutScaling=2^0  OutDataTypeStr=uint8
  receiver_net_address : Inport  Tag=id=_rYX9sPdmEeGH_6eRdlYQdA  Port=3  PortDimensions=-1  DataType=uint8  OutDataType=fixdt(1, 16)  OutScaling=2^0  OutDataTypeStr=uint8
  read_event_queue_in : Inport  Tag=id=_rYPa0PdmEeGH_6eRdlYQdA  Port=4  PortDimensions=-1  DataType=auto  OutDataType=fixdt(1, 16)  OutScaling=2^0  OutDataTypeStr=Inherit: auto
  read_event_param_queue_in : Inport  Tag=id=_rYRQAPdmEeGH_6eRdlYQdA  Port=5  PortDimensions=-1  DataType=auto  OutDataType=fixdt(1, 16)  OutScaling=2^0  OutDataTypeStr=Inherit: auto
  read_event_queue_out : Inport  Tag=id=_rYSeIPdmEeGH_6eRdlYQdA  Port=6  PortDimensions=-1  DataType=auto  OutDataType=fixdt(1, 16)  OutScaling=2^0  OutDataTypeStr=Inherit: auto
  read_event_param_queue_out : Inport  Tag=id=_rYTsQPdmEeGH_6eRdlYQdA  Port=7  PortDimensions=-1  DataType=auto  OutDataType=fixdt(1, 16)  OutScaling=2^0  OutDataTypeStr=Inherit: auto
  port_out : Outport  Tag=id=_rYOMsPdmEeGH_6eRdlYQdA  Port=1  PortDimensions=-1  DataType=auto  OutDataType=fixdt(1, 16)  OutScaling=2^0  UseBusObject=on  OutDataTypeStr=Inherit: auto
      settings: BusObject=PacketBus
  write_event_queue_in : Outport  Tag=id=_rYQB4PdmEeGH_6eRdlYQdA  Port=2  PortDimensions=-1  DataType=auto  OutDataType=fixdt(1, 16)  OutScaling=2^0  OutDataTypeStr=Inherit: auto
  write_event_param_queue_in : Outport  Tag=id=_rYQo8PdmEeGH_6eRdlYQdA  Port=3  PortDimensions=-1  DataType=auto  OutDataType=fixdt(1, 16)  OutScaling=2^0  OutDataTypeStr=Inherit: auto
  write_event_queue_out : Outport  Tag=id=_rYUTUPdmEeGH_6eRdlYQdA  Port=4  PortDimensions=-1  DataType=auto  OutDataType=fixdt(1, 16)  OutScaling=2^0  OutDataTypeStr=Inherit: auto
  write_event_param_queue_out : Outport  Tag=id=_rYVhcPdmEeGH_6eRdlYQdA  Port=5  PortDimensions=-1  DataType=auto  OutDataType=fixdt(1, 16)  OutScaling=2^0  OutDataTypeStr=Inherit: auto
  DataLinkLayer : Subsystem  Tag=id=_rYZy4fdmEeGH_6eRdlYQdA
  Bus Selector : BusSelector  OutputSignals=from,to,msg,param,pkgid,time  Tag=id=_rYZL0PdmEeGH_6eRdlYQdA
  Unit Delay1 : UnitDelay  Tag=id=_rYZL0fdmEeGH_6eRdlYQdA  SampleTime=-1
  Unit Delay2 : UnitDelay  Tag=id=_rYZy4PdmEeGH_6eRdlYQdA  SampleTime=-1
  Unit Delay3 : UnitDelay  Tag=id=_rYaZ8PdmEeGH_6eRdlYQdA  SampleTime=-1
  Bus Creator : BusCreator  Inputs=6  UseBusObject=on  Tag=id=_rYbBAPdmEeGH_6eRdlYQdA
      settings: BusObject=PacketBus
  Unit Delay4 : UnitDelay  Tag=id=_rYbBAfdmEeGH_6eRdlYQdA  SampleTime=-1
  Terminator : Terminator
      settings: Tag=id=_rYboEPdmEeGH_6eRdlYQdA
  Receive Packet : Stateflow chart  Tag=id=_rYboEfdmEeGH_6eRdlYQdA
  Send Packet : Stateflow chart  Tag=id=_rYcPIPdmEeGH_6eRdlYQdA
  wires:
  DataLinkLayer/3(snd_msg_out) -> Bus Creator/3
  DataLinkLayer/8(recv_msg_out) -> Receive Packet/2(packetMsg)
  Send Packet/3(eventQueue) -> Unit Delay1/1
  DataLinkLayer/7(recv_from_out) -> Receive Packet/1(packetFrom)
  Bus Selector/3 -> DataLinkLayer/3(recv_msg_in)
  read_event_param_queue_in/1 -> Receive Packet/5(eventParamQueueIn)
  Receive Packet/3(bufferOverflow) -> Terminator/1
  receiver_net_address/1 -> DataLinkLayer/8(snd_to_in)
  Receive Packet/2(eventParamQueue) -> Unit Delay4/1
  read_event_queue_out/1 -> Send Packet/2(eventQueueIn)
  DataLinkLayer/9(recv_param_out) -> Receive Packet/3(packetParam)
  Send Packet/2(packetParam) -> DataLinkLayer/10(snd_param_in)
  Bus Selector/2 -> DataLinkLayer/2(recv_to_in)
  port_in/1 -> Bus Selector/1
  read_event_param_queue_out/1 -> Send Packet/3(eventParamQueueIn)
  Send Packet/4(eventParamQueue) -> Unit Delay2/1
  Bus Selector/5 -> DataLinkLayer/5(recv_pkgid_in)
  Unit Delay4/1 -> write_event_param_queue_in/1
  read_event_queue_in/1 -> Receive Packet/4(eventQueueIn)
  Bus Selector/4 -> DataLinkLayer/4(recv_param_in)
  DataLinkLayer/2(snd_to_out) -> Bus Creator/2
  Bus Selector/6 -> DataLinkLayer/6(recv_time_in), Send Packet/1(busSizeSignal)
  Receive Packet/1(eventQueue) -> Unit Delay3/1
  DataLinkLayer/6(snd_time_out) -> Bus Creator/6
  Unit Delay1/1 -> write_event_queue_out/1
  DataLinkLayer/1(snd_from_out) -> Bus Creator/1
  DataLinkLayer/5(snd_pkgid_out) -> Bus Creator/5
  net_address/1 -> DataLinkLayer/7(snd_from_in)
  Send Packet/1(packetMsg) -> DataLinkLayer/9(snd_msg_in)
  Bus Creator/1 -> port_out/1  "Outport33"
  Unit Delay3/1 -> write_event_queue_in/1
  Bus Selector/1 -> DataLinkLayer/1(recv_from_in)
  Unit Delay2/1 -> write_event_param_queue_out/1
  DataLinkLayer/4(snd_param_out) -> Bus Creator/4

== system AtomicLibrary/TestStartStopSlave/Link Layer startStop_Slave ==
  port_in : Inport  Tag=id=_rhBjYPdmEeGH_6eRdlYQdA  Port=1  PortDimensions=-1  DataType=auto  OutDataType=fixdt(1, 16)  OutScaling=2^0  UseBusObject=on  OutDataTypeStr=Inherit: auto
      settings: BusObject=PacketBus
  net_address : Inport  Tag=id=_rhHqAPdmEeGH_6eRdlYQdA  Port=2  PortDimensions=-1  DataType=uint8  OutDataType=fixdt(1, 16)  OutScaling=2^0  OutDataTypeStr=uint8
  receiver_net_address : Inport  Tag=id=_rhI4IPdmEeGH_6eRdlYQdA  Port=3  PortDimensions=-1  DataType=uint8  OutDataType=fixdt(1, 16)  OutScaling=2^0  OutDataTypeStr=uint8
  read_event_queue_in : Inport  Tag=id=_rhCKcPdmEeGH_6eRdlYQdA  Port=4  PortDimensions=-1  DataType=auto  OutDataType=fixdt(1, 16)  OutScaling=2^0  OutDataTypeStr=Inherit: auto
  read_event_param_queue_in : Inport  Tag=id=_rhD_oPdmEeGH_6eRdlYQdA  Port=5  PortDimensions=-1  DataType=auto  OutDataType=fixdt(1, 16)  OutScaling=2^0  OutDataTypeStr=Inherit: auto
  read_event_queue_out : Inport  Tag=id=_rhFNwPdmEeGH_6eRdlYQdA  Port=6  PortDimensions=-1  DataType=auto  OutDataType=fixdt(1, 16)  OutScaling=2^0  OutDataTypeStr=Inherit: auto
  read_event_param_queue_out : Inport  Tag=id=_rhF00PdmEeGH_6eRdlYQdA  Port=7  PortDimensions=-1  DataType=auto  OutDataType=fixdt(1, 16)  OutScaling=2^0  OutDataTypeStr=Inherit: auto
  port_out : Outport  Tag=id=_rhA8UfdmEeGH_6eRdlYQdA  Port=1  PortDimensions=-1  DataType=auto  OutDataType=fixdt(1, 16)  OutScaling=2^0  UseBusObject=on  OutDataTypeStr=Inherit: auto
      settings: BusObject=PacketBus
  write_event_queue_in : Outport  Tag=id=_rhCxgPdmEeGH_6eRdlYQdA  Port=2  PortDimensions=-1  DataType=auto  OutDataType=fixdt(1, 16)  OutScaling=2^0  OutDataTypeStr=Inherit: auto
  write_event_param_queue_in : Outport  Tag=id=_rhDYkPdmEeGH_6eRdlYQdA  Port=3  PortDimensions=-1  DataType=auto  OutDataType=fixdt(1, 16)  OutScaling=2^0  OutDataTypeStr=Inherit: auto
  write_event_queue_out : Outport  Tag=id=_rhGb4PdmEeGH_6eRdlYQdA  Port=4  PortDimensions=-1  DataType=auto  OutDataType=fixdt(1, 16)  OutScaling=2^0  OutDataTypeStr=Inherit: auto
  write_event_param_queue_out : Outport  Tag=id=_rhHC8PdmEeGH_6eRdlYQdA  Port=5  PortDimensions=-1  DataType=auto  OutDataType=fixdt(1, 16)  OutScaling=2^0  OutDataTypeStr=Inherit: auto
  DataLinkLayer : Subsystem  Tag=id=_rhKGQfdmEeGH_6eRdlYQdA
  Bus Selector : BusSelector  OutputSignals=from,to,msg,param,pkgid,time  Tag=id=_rhJfMPdmEeGH_6eRdlYQdA
  Unit Delay1 : UnitDelay  Tag=id=_rhJfMfdmEeGH_6eRdlYQdA  SampleTime=-1
  Unit Delay2 : UnitDelay  Tag=id=_rhKGQPdmEeGH_6eRdlYQdA  SampleTime=-1
  Unit Delay3 : UnitDelay  Tag=id=_rhKtUPdmEeGH_6eRdlYQdA  SampleTime=-1
  Bus Creator : BusCreator  Inputs=6  UseBusObject=on  Tag=id=_rhKtUfdmEeGH_6eRdlYQdA
      settings: BusObject=PacketBus
  Unit Delay4 : UnitDelay  Tag=id=_rhKtUvdmEeGH_6eRdlYQdA  SampleTime=-1
  Terminator : Terminator
      settings: Tag=id=_rhLUYPdmEeGH_6eRdlYQdA
  Receive Packet : Stateflow chart  Tag=id=_rhLUYfdmEeGH_6eRdlYQdA
  Send Packet : Stateflow chart  Tag=id=_rhL7cPdmEeGH_6eRdlYQdA
  wires:
  DataLinkLayer/3(snd_msg_out) -> Bus Creator/3
  DataLinkLayer/8(recv_msg_out) -> Receive Packet/2(packetMsg)
  Send Packet/3(eventQueue) -> Unit Delay1/1
  DataLinkLayer/7(recv_from_out) -> Receive Packet/1(packetFrom)
  Bus Selector/3 -> DataLinkLayer/3(recv_msg_in)
  read_event_param_queue_in/1 -> Receive Packet/5(eventParamQueueIn)
  Receive Packet/3(bufferOverflow) -> Terminator/1
  receiver_net_address/1 -> DataLinkLayer/8(snd_to_in)
  Receive Packet/2(eventParamQueue) -> Unit Delay4/1
  read_event_queue_out/1 -> Send Packet/2(eventQueueIn)
  DataLinkLayer/9(recv_param_out) -> Receive Packet/3(packetParam)
  Send Packet/2(packetParam) -> DataLinkLayer/10(snd_param_in)
  Bus Selector/2 -> DataLinkLayer/2(recv_to_in)
  port_in/1 -> Bus Selector/1
  read_event_param_queue_out/1 -> Send Packet/3(eventParamQueueIn)
  Send Packet/4(eventParamQueue) -> Unit Delay2/1
  Bus Selector/5 -> DataLinkLayer/5(recv_pkgid_in)
  Unit Delay4/1 -> write_event_param_queue_in/1
  read_event_queue_in/1 -> Receive Packet/4(eventQueueIn)
  Bus Selector/4 -> DataLinkLayer/4(recv_param_in)
  DataLinkLayer/2(snd_to_out) -> Bus Creator/2
  Bus Selector/6 -> DataLinkLayer/6(recv_time_in), Send Packet/1(busSizeSignal)
  Receive Packet/1(eventQueue) -> Unit Delay3/1
  DataLinkLayer/6(snd_time_out) -> Bus Creator/6
  Unit Delay1/1 -> write_event_queue_out/1
  DataLinkLayer/1(snd_from_out) -> Bus Creator/1
  DataLinkLayer/5(snd_pkgid_out) -> Bus Creator/5
  net_address/1 -> DataLinkLayer/7(snd_from_in)
  Send Packet/1(packetMsg) -> DataLinkLayer/9(snd_msg_in)
  Bus Creator/1 -> port_out/1  "Outport35"
  Unit Delay3/1 -> write_event_queue_in/1
  Bus Selector/1 -> DataLinkLayer/1(recv_from_in)
  Unit Delay2/1 -> write_event_param_queue_out/1
  DataLinkLayer/4(snd_param_out) -> Bus Creator/4
